simulink model "SynchronousExample"  (R2023a)
settings: Solver=VariableStepAuto  StartTime=0.0  StopTime=10.0  RelTol=1e-3
settings Model: Creator=Administrator  LastModifiedBy=wkmiao
settings RTWCC: GPUComputeCapability=5.0

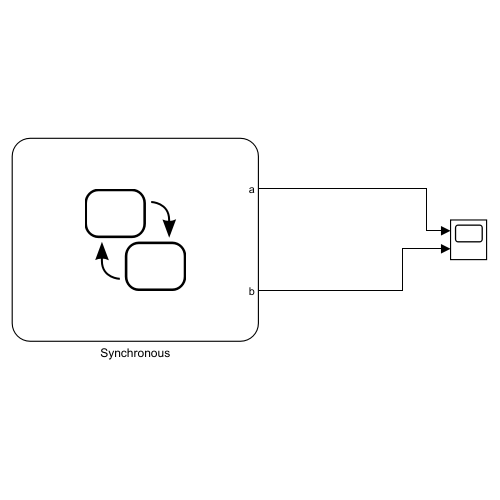
[thumbnail: Simulink's stored preview of the top-level diagram]
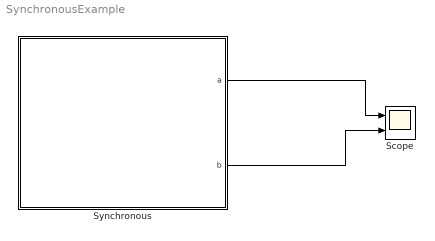
== system SynchronousExample ==
  Scope : Scope  NumInputPorts=2
  Synchronous : Stateflow chart  TreatAsAtomicUnit=on
  wires:
  Synchronous/1(a) -> Scope/1
  Synchronous/2(b) -> Scope/2

== stateflow chart SynchronousExample/Synchronous ==
  settings: initializeOutput=1
  state outputa [parallel]
    settings: executionOrder=1
    state s1
    state s2
    (default) -> s1
    s1 -> s2 : {a = 1}
    s2 -> s1
  state outputb [parallel]
    settings: executionOrder=2
    state s3
    state s4
    (default) -> s3
    s3 -> s4
    s4 -> s3 : {b = 2}
  data: a output; b output
